simulink model "PID"  (R2023b)
settings: Solver=VariableStepAuto  StartTime=0.0  StopTime=10.0  RelTol=1e-3
values from neighbouring files (symbols this model uses):
  b_a = J_eq*(2*zeta+1)*wp    (= 0.0395694444444)    [parametros.m]
  K_sa = J_eq*(2*zeta+1)*wp^2    (= 31.6555555556)    [parametros.m]
  K_sia = J_eq*wp^3    (= 10129.7777778)    [parametros.m]
settings Model: Creator=AAgus  LastModifiedBy=Marti

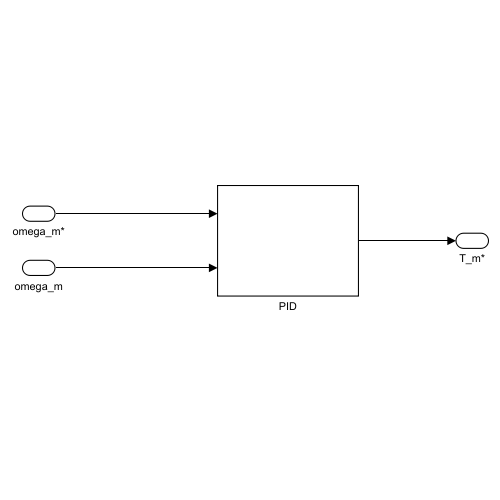
[thumbnail: Simulink's stored preview of the top-level diagram]
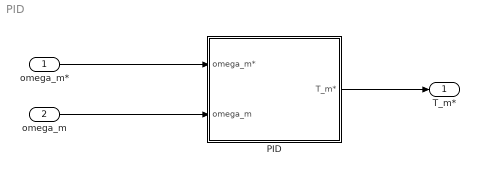
== system PID ==
  omega_m* : Inport
  omega_m : Inport  Port=2
  PID : Subsystem
  T_m* : Outport
  wires:
  omega_m*/1 -> PID/1(omega_m*)
  omega_m/1 -> PID/2(omega_m)
  PID/1(T_m*) -> T_m*/1

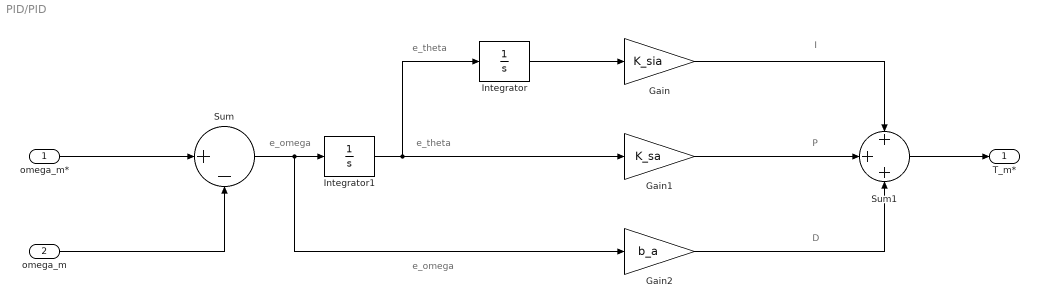
== system PID/PID ==
  note: e_theta
  note: e_omega
  note: e_theta
  note: e_omega
  note: I
  note: P
  note: D
  omega_m* : Inport
  omega_m : Inport  Port=2
  Gain : Gain  Gain=K_sia
  Gain1 : Gain  Gain=K_sa
  Gain2 : Gain  Gain=b_a
  Integrator : Integrator
  Integrator1 : Integrator
  Sum : Sum  Inputs=|+-
  Sum1 : Sum  Inputs=+++
  T_m* : Outport
  wires:
  Gain2/1 -> Sum1/3
  Gain1/1 -> Sum1/2
  Integrator1/1 -> Gain1/1, Integrator/1
  Sum1/1 -> T_m*/1
  omega_m/1 -> Sum/2
  Gain/1 -> Sum1/1
  Integrator/1 -> Gain/1
  omega_m*/1 -> Sum/1
  Sum/1 -> Gain2/1, Integrator1/1
